simulink model "mic_input"  (R2013b)
settings: Solver=FixedStepDiscrete  StartTime=0.0  StopTime=3  FixedStep=1/44100  RelTol=1e-3
libraries: dspsrcs4 x5
settings Model: Creator=nryan1_guest  LastModifiedBy=nryan1_guest

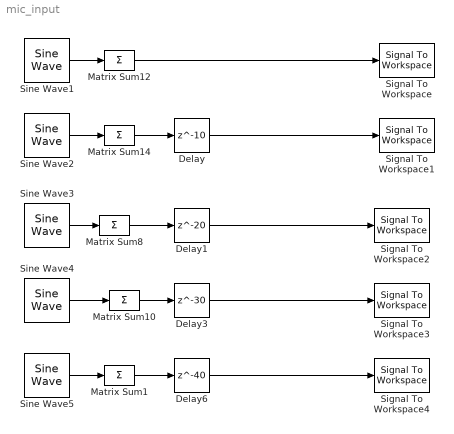
== system mic_input ==
  Delay : Delay  DelayLength=10  InitialCondition=0
  Delay1 : Delay  DelayLength=20  InitialCondition=0
  Delay3 : Delay  DelayLength=30  InitialCondition=0
  Delay6 : Delay  DelayLength=40  InitialCondition=0
  Matrix Sum{1,8,10,12,14} (5 alike) : Sum  Inputs=+  CollapseMode=Specified dimension  CollapseDim=2  SampleTime=1/44100
  Signal To Workspace : SignalToWorkspace  VariableName=mic1
      settings: CopyFcn=dspblkcopystw(gcbh);
  Signal To Workspace1 : SignalToWorkspace  VariableName=mic2
      settings: CopyFcn=dspblkcopystw(gcbh);
  Signal To Workspace2 : SignalToWorkspace  VariableName=mic3
      settings: CopyFcn=dspblkcopystw(gcbh);
  Signal To Workspace3 : SignalToWorkspace  VariableName=mic4
      settings: CopyFcn=dspblkcopystw(gcbh);
  Signal To Workspace4 : SignalToWorkspace  VariableName=mic5
      settings: CopyFcn=dspblkcopystw(gcbh);
  Sine Wave{1..5} (5 alike) : dspsrcs4/Sine Wave  Amplitude=5  Frequency=440  Phase=0  SampleMode=Discrete  OutComplex=Real  CompMethod=Trigonometric fcn  TableSize=Speed  SampleTime=1/44100  SamplesPerFrame=1  ResetState=Restart at time zero  dataType=double  wordLen=16  udDataType=sfix(16)  fracBitsMode=Best precision  numFracBits=15  OutDataTypeStr=double  LastOutDataTypeStr=double
  wires:
  Sine Wave1/1 -> Matrix Sum12/1
  Sine Wave3/1 -> Matrix Sum8/1
  Sine Wave2/1 -> Matrix Sum14/1
  Matrix Sum14/1 -> Delay/1
  Matrix Sum8/1 -> Delay1/1
  Sine Wave4/1 -> Matrix Sum10/1
  Matrix Sum10/1 -> Delay3/1
  Matrix Sum12/1 -> Signal To Workspace/1
  Delay3/1 -> Signal To Workspace3/1
  Delay1/1 -> Signal To Workspace2/1
  Delay/1 -> Signal To Workspace1/1
  Sine Wave5/1 -> Matrix Sum1/1
  Matrix Sum1/1 -> Delay6/1
  Delay6/1 -> Signal To Workspace4/1
